simulink model "sfcndemo_mixedmex"  (Simulink 7.6)
settings: Solver=ode5  SolverMode=SingleTasking  StartTime=0.0  StopTime=10.0  FixedStep=.01  RelTol=1e-3
Description:
  | Mixed Continuous and Discrete States Dynamic System C-MEX S-function
settings Model: Creator=The MathWorks Inc.  ExtModeTrigMode=oneshot  ExtModeArmWhenConnect=off  ExtModeAutoUpdateStatusClock=off
settings DataIOCC: LimitDataPoints=off
settings OptimizationCC: BlockReduction=off  BooleanDataType=off  InitFltsAndDblsToZero=on
settings DebuggingCC: SaveWithParameterizedLinksMsg=none  SignalResolutionControl=TryResolveAllWithWarning  SolverPrmCheckMsg=none  MultiTaskDSMMsg=warning  MultiTaskCondExecSysMsg=none
settings HardwareCC: TargetUnknown=on
settings RTWCC: IncludeERTFirstTime=on
settings CodeAppCC: CustomSymbolStrFcn=$F$N$M
settings GRTTargetCC: TargetFcnLib=ansi_tfl_tmw.mat

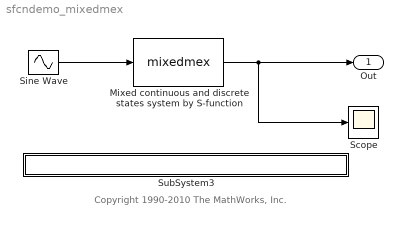
== system sfcndemo_mixedmex ==
  note: Copyright 1990-2010 The MathWorks, Inc.
  Mixed continuous and discrete states system by S-function : S-Function  FunctionName=mixedmex  EnableBusSupport=off
      mask Type: S-function: mixedmex
      mask Description: A single-input, single-output system with mixed continuous and discrete states by a S-function.
      mask Display: disp('Single Input\nSingle Output');
  Scope : Scope
      settings: TimeRange=10  YMin=1  YMax=3
  Sine Wave : Sin  SampleTime=0
  SubSystem3 : Subsystem  mask{filename=mixedmex.c}
      mask init:
      | x=sfundemo_maskdisp;
      settings: AttributesFormatString=\n  OpenFcn=sfundemo_openfcn
      mask Display: disp(x);
  Out : Outport  InitialOutput=0
  wires:
  Sine Wave/1 -> Mixed continuous and discrete states system by S-function/1
  Mixed continuous and discrete states system by S-function/1 -> Out/1, Scope/1

== system sfcndemo_mixedmex/SubSystem3 ==
